simulink model "s_msd"  (R2017b)
settings: Solver=VariableStepAuto  StartTime=0.0  StopTime=10.0  RelTol=1e-3
values from neighbouring files (symbols this model uses):
  b = randi([1,1e1])    [EGH445_Computer_Lab_1.m]    (also in mass_spring_damper_script.m = 1; sim_msd_diff_solvers.m = 100)
  c = 1    [sim_msd_diff_solvers.m]
  m = 0.15    [CP_ContrSys_Lin_a_Mainfile_n9329013.m]    (also in CP_ContrSys_Lin_b_Mainfile_n9329013.m; MainFile_9329013.m; MainFile_Linearised_a_9329013.m; MainFile_Linearised_b_9329013.m)
settings Model: Creator=Koh Kim Hai  LastModifiedBy=Koh Kim Hai

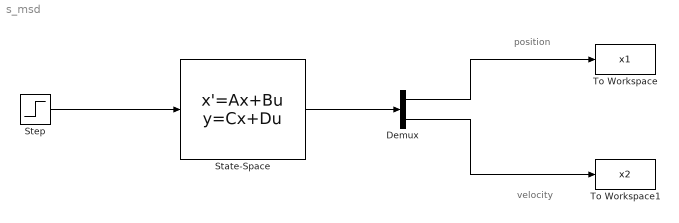
== system s_msd ==
  note: velocity
  note: position
  Demux : Demux  Outputs=2
  State-Space : StateSpace  A=[0,1;(-1/(c*m)),(-b/m)]  B=[0;1/m]  C=[1,0;0,1]  D=[0;0]  InitialCondition=0
  Step : Step  SampleTime=0
  To Workspace : ToWorkspace  VariableName=x1  SampleTime=-1
  To Workspace1 : ToWorkspace  VariableName=x2  SampleTime=-1
  wires:
  State-Space/1 -> Demux/1
  Demux/1 -> To Workspace/1
  Demux/2 -> To Workspace1/1
  Step/1 -> State-Space/1
